simulink model "exp3_3_sim"  (R2023b)
settings: Solver=VariableStepAuto  StartTime=0.0  StopTime=10.0  RelTol=1e-3
settings Model: Creator=Paljoy  LastModifiedBy=27198
settings DataIOCC: ReturnWorkspaceOutputs=off

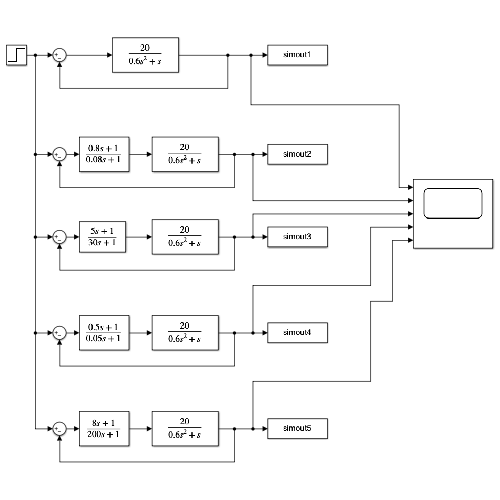
[thumbnail: Simulink's stored preview of the top-level diagram]
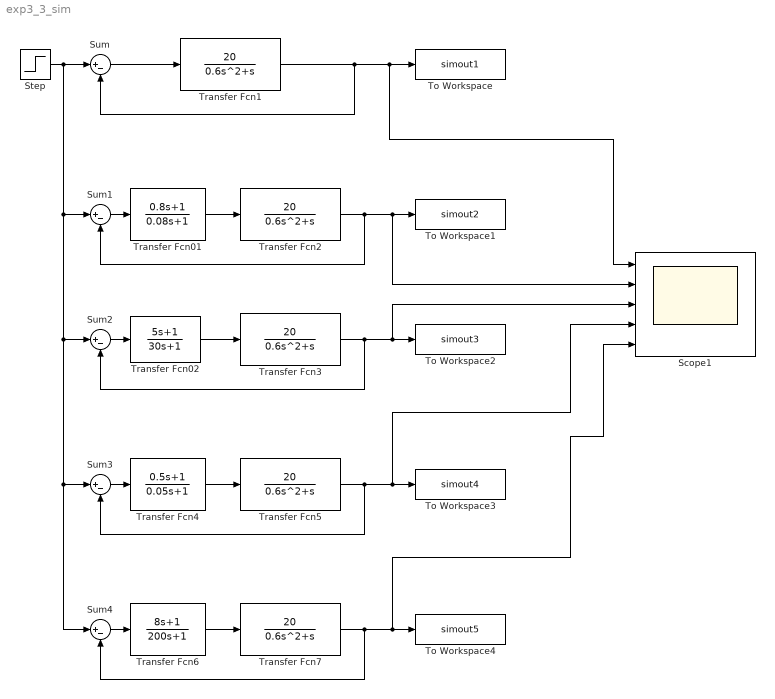
== system exp3_3_sim ==
  Scope1 : Scope  NumInputPorts=5
  Step : Step  SampleTime=0
  Sum{,1..4} (5 alike) : Sum  Inputs=|+-
  To Workspace : ToWorkspace  VariableName=simout1  SaveFormat=Timeseries  SampleTime=0.01
  To Workspace1 : ToWorkspace  VariableName=simout2  SaveFormat=Timeseries  SampleTime=0.01
  To Workspace2 : ToWorkspace  VariableName=simout3  SaveFormat=Timeseries  SampleTime=0.01
  To Workspace3 : ToWorkspace  VariableName=simout4  SaveFormat=Timeseries  SampleTime=0.01
  To Workspace4 : ToWorkspace  VariableName=simout5  SaveFormat=Timeseries  SampleTime=0.01
  Transfer Fcn01 : TransferFcn  Numerator=[0.8 1]  Denominator=[0.08 1]
  Transfer Fcn02 : TransferFcn  Numerator=[5 1]  Denominator=[30 1]
  Transfer Fcn{1..3,5,7} (5 alike) : TransferFcn  Numerator=[20]  Denominator=[0.6 1 0]
  Transfer Fcn4 : TransferFcn  Numerator=[0.5 1]  Denominator=[0.05 1]
  Transfer Fcn6 : TransferFcn  Numerator=[8 1]  Denominator=[200 1]
  wires:
  Transfer Fcn01/1 -> Transfer Fcn2/1
  Transfer Fcn02/1 -> Transfer Fcn3/1
  Sum/1 -> Transfer Fcn1/1
  Sum2/1 -> Transfer Fcn02/1
  Transfer Fcn1/1 -> Sum/2, Scope1/1, To Workspace/1
  Transfer Fcn2/1 -> Scope1/2, To Workspace1/1, Sum1/2
  Transfer Fcn3/1 -> Sum2/2, Scope1/3, To Workspace2/1
  Sum1/1 -> Transfer Fcn01/1
  Sum3/1 -> Transfer Fcn4/1
  Transfer Fcn5/1 -> Sum3/2, Scope1/4, To Workspace3/1
  Step/1 -> Sum1/1, Sum4/1, Sum3/1, Sum2/1, Sum/1
  Transfer Fcn4/1 -> Transfer Fcn5/1
  Transfer Fcn6/1 -> Transfer Fcn7/1
  Transfer Fcn7/1 -> To Workspace4/1, Scope1/5, Sum4/2
  Sum4/1 -> Transfer Fcn6/1
